simulink model "velocity_control"  (R2022b)
settings: Solver=FixedStepAuto  StartTime=0.0  StopTime=inf  FixedStep=0.05  RelTol=1e-3
undefined symbols (not defined in the file): Angular, Linear
libraries: robotlib x6
settings Model: Creator=refulgent  LastModifiedBy=refulgent
settings OptimizationCC: EnhancedBackFolding=on  PassReuseOutputArgsAs=Individual arguments  ZeroExternalMemoryAtStartup=off  ZeroInternalMemoryAtStartup=off  MaxStackSize=64  OptimizeBlockOrder=speed  DifferentSizesBufferReuse=on  OptimizationCustomize=off  EfficientTunableParamExpr=on
settings DebuggingCC: ParameterTunabilityLossMsg=error
settings HardwareCC: ProdBitPerPointer=32  ProdBitPerSizeT=32  ProdBitPerPtrDiffT=32  ProdLargestAtomicFloat=None  ProdIntDivRoundTo=Undefined  ProdEndianess=Unspecified  ProdWordSize=32  ProdHWDeviceType=Generic->Unspecified (assume 32-bit Generic)
settings SFSimCC: MATLABDynamicMemAlloc=off
settings RTWCC: Description=Embedded Coder  SystemTargetFile=ert.tlc  HardwareBoard=Robot Operating System (ROS)  TLCOptions="-aInlineSetEventsForThisBaseRateFcn=TLC_FALSE -aSuppressMultiTaskScheduler=TLC_FALSE  -aRateBasedStepFcn=0"  TemplateMakefile=ert_default_tmf  Toolchain=Catkin  TargetLang=C++
settings CodeAppCC: ForceParamTrailComments=on  IgnoreCustomStorageClasses=off  OperatorAnnotations=on  SimulinkDataObjDesc=on  SFDataObjDesc=on  InsertBlockDesc=on

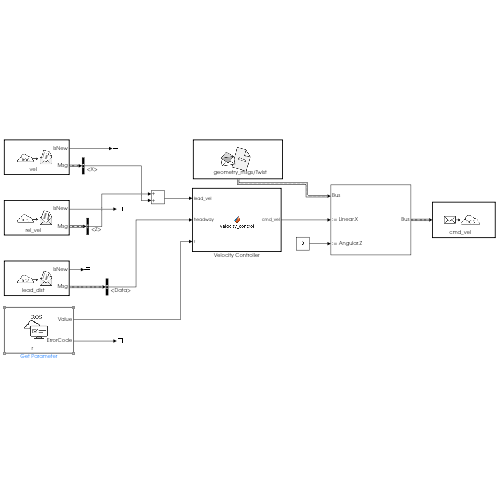
[thumbnail: Simulink's stored preview of the top-level diagram]
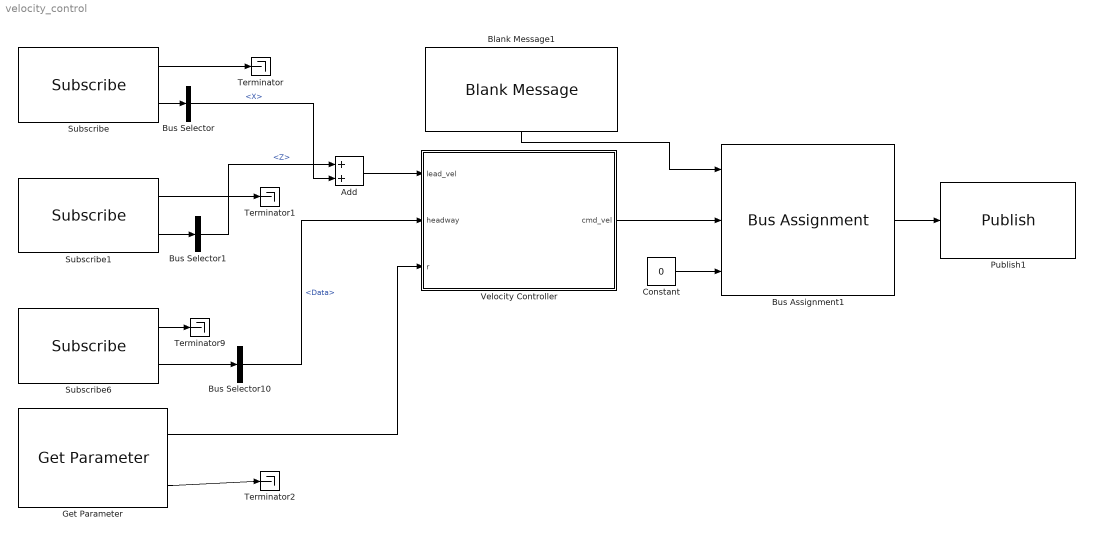
== system velocity_control ==
  Add : Sum
  Blank Message1 : robotlib/Blank Message  messageClass=Message  entityType=geometry_msgs/Twist  messageType=geometry_msgs/Twist  SampleTime=inf  legacyBusStruct=off
  Bus Assignment1 : BusAssignment  AssignedSignals=Linear.X,Angular.Z
  Bus Selector : BusSelector  OutputSignals=Linear.X
  Bus Selector1 : BusSelector  OutputSignals=Linear.Z
  Bus Selector10 : BusSelector  OutputSignals=Data
  Constant : Constant  Value=0
  Get Parameter : robotlib/Get Parameter  ParameterSource=Specify your own  ParameterName=r  ParameterType=double  ParameterMaxArrayLength=16  ParameterInitialValue=20.0  SampleTime=-1  ShowErrorCodeOutput=on  ModelName=velocity_control  BlockId=ParamGet_velocity_control_21
  Publish1 : robotlib/Publish  topicSource=Specify your own  topic=cmd_vel  messageType=geometry_msgs/Twist  legacyBusStruct=off  messageQueueLength=1
  Subscribe : robotlib/Subscribe  topicSource=Specify your own  topic=vel  messageType=geometry_msgs/Twist  SampleTime=-1  legacyBusStruct=off  messageQueueLength=1
      settings: LibrarySourceBlock=roslib/ROS/Subscribe
  Subscribe1 : robotlib/Subscribe  topicSource=Specify your own  topic=rel_vel  messageType=geometry_msgs/Twist  SampleTime=-1  legacyBusStruct=off  messageQueueLength=1
      settings: LibrarySourceBlock=roslib/ROS/Subscribe
  Subscribe6 : robotlib/Subscribe  topicSource=Specify your own  topic=lead_dist  messageType=std_msgs/Float64  SampleTime=-1  legacyBusStruct=off  messageQueueLength=1
  Terminator{,1..2,9} (4 alike) : Terminator
  Velocity Controller : MATLAB Function  TreatAsAtomicUnit=on
  wires:
  Subscribe/1 -> Terminator/1
  Subscribe/2 -> Bus Selector/1
  Subscribe1/2 -> Bus Selector1/1
  Subscribe1/1 -> Terminator1/1
  Subscribe6/1 -> Terminator9/1
  Subscribe6/2 -> Bus Selector10/1
  Bus Selector/1 -> Add/2  "<X>"
  Bus Selector1/1 -> Add/1  "<Z>"
  Bus Selector10/1 -> Velocity Controller/2(headway)  "<Data>"
  Get Parameter/1 -> Velocity Controller/3(r)
  Get Parameter/2 -> Terminator2/1
  Add/1 -> Velocity Controller/1(lead_vel)
  Bus Assignment1/1 -> Publish1/1
  Blank Message1/1 -> Bus Assignment1/1
  Constant/1 -> Bus Assignment1/3
  Velocity Controller/1(cmd_vel) -> Bus Assignment1/2

== matlab function velocity_control/Velocity Controller ==
  data: cmd_vel output; lead_vel input; headway input; r input
function cmd_vel = velocity_control(lead_vel, headway, r)


if(headway > 30)
    cmd_vel = r + 0.5*lead_vel;
elseif(headway == 30)
    cmd_vel = r;
else
    cmd_vel = r - 0.5*lead_vel;
end
